simulink model "mm_autograde_M1"  (R2025a)
settings: Solver=FixedStepAuto  StartTime=0.0  StopTime=30  FixedStep=0.005  RelTol=1e-3
libraries: mmuct_lib x2
settings Model: PacingRate=2  Creator=nicolls  LastModifiedBy=MTMTAD006
settings RTWCC: GenCodeOnly=on

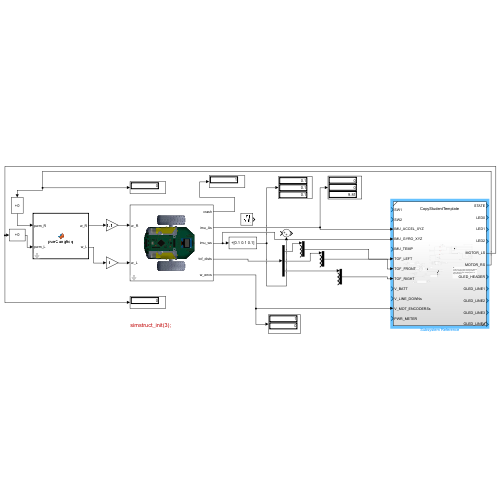
[thumbnail: Simulink's stored preview of the top-level diagram]
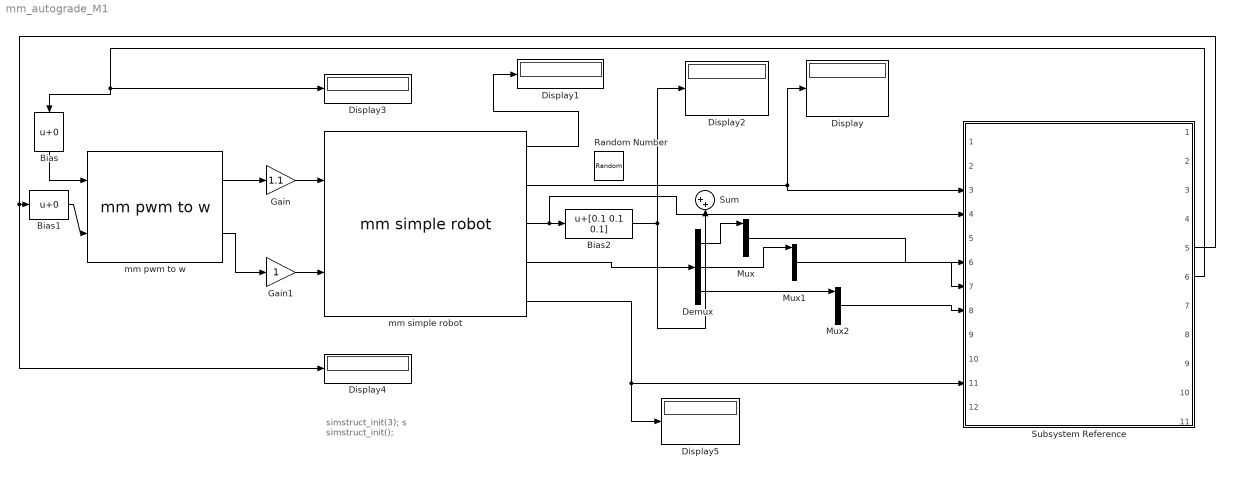
== system mm_autograde_M1 ==
  note: simstruct_init(3);
      | s
      | simstruct_init();
  Bias : Bias  SaturateOnIntegerOverflow=off
  Bias1 : Bias  SaturateOnIntegerOverflow=off
  Bias2 : Bias  Bias=[0.1 0.1 0.1]  SaturateOnIntegerOverflow=off
  Demux : Demux  Outputs=3
  Display{,1..5} (6 alike) : Display
  Gain : Gain  Gain=1.1
  Gain1 : Gain
  Mux : Mux
  Mux1 : Mux
  Mux2 : Mux
  Random Number : RandomNumber  SampleTime=0.1
  Subsystem Reference : Subsystem  ReferencedSubsystem=CopyStudentTemplate
  Sum : Sum  Inputs=|++
  mm pwm to w : mmuct_lib/mm pwm to w  deadb=0  maxw=2*pi  motd=0
  mm simple robot : mmuct_lib/mm simple robot  simstruct=simstruct  x0=0.3  y0=0.75  theta0=0
      settings: SourceProductName=UCT EEE Micromouse
  wires:
  Demux/1 -> Mux/1
  Demux/2 -> Mux1/1
  Demux/3 -> Mux2/1
  Subsystem Reference/6 -> Display3/1, Bias/1
  mm simple robot/3 -> Subsystem Reference/4, Bias2/1
  mm simple robot/1 -> Display1/1
  mm simple robot/5 -> Display5/1, Subsystem Reference/11
  mm pwm to w/2 -> Gain1/1
  mm pwm to w/1 -> Gain/1
  Mux2/1 -> Subsystem Reference/8
  Mux1/1 -> Subsystem Reference/7
  Mux/1 -> Subsystem Reference/6
  mm simple robot/2 -> Display/1, Subsystem Reference/3
  Subsystem Reference/5 -> Bias1/1, Display4/1
  mm simple robot/4 -> Demux/1
  Gain/1 -> mm simple robot/1
  Gain1/1 -> mm simple robot/2
  Bias/1 -> mm pwm to w/1
  Bias1/1 -> mm pwm to w/2
  Bias2/1 -> Display2/1, Sum/2
